simulink model "untitled"  (R2023b)
settings: Solver=ode4  StartTime=0.0  StopTime=100  FixedStep=.02  RelTol=1e-3
values from neighbouring files (symbols this model uses):
  allocation_matrix = [ -0.418379550895652   0.707106781186547   1.000000000000000  -1 ... (first row only)    [Octa_Copter_Parameters.m]
  b_m = 1.645552813e-3    (= 0.001645552813)    [Octa_Copter_Parameters.m]
  d_m = 2.6675567e-3    (= 0.0026675567)    [Octa_Copter_Parameters.m]
  g = 9.81    [Octa_Copter_Parameters.m]
  lx1 = 0.47    [Octa_Copter_Parameters.m]
  lx2 = 0.47    [Octa_Copter_Parameters.m]
  lx3 = 0.47    [Octa_Copter_Parameters.m]
  lx4 = lx1    (= 0.47)    [Octa_Copter_Parameters.m]
  lx5 = 0.47    [Octa_Copter_Parameters.m]
  lx6 = 0.47    [Octa_Copter_Parameters.m]
  lx7 = 0.47    [Octa_Copter_Parameters.m]
  lx8 = lx5    (= 0.47)    [Octa_Copter_Parameters.m]
  ly1 = 0.255    [Octa_Copter_Parameters.m]
  ly2 = 0.255    [Octa_Copter_Parameters.m]
  ly3 = 0.255    [Octa_Copter_Parameters.m]
  ly4 = 0.255    [Octa_Copter_Parameters.m]
  ly5 = 0.548    [Octa_Copter_Parameters.m]
  ly6 = 0.548    [Octa_Copter_Parameters.m]
  ly7 = 0.548    [Octa_Copter_Parameters.m]
  ly8 = 0.548    [Octa_Copter_Parameters.m]
  m = 4.455    [Octa_Copter_Parameters.m]
  omega_nom = sqrt((m*g)/(8*b_m))    [Octa_Copter_Parameters.m]
undefined symbols (not defined in the file or in its folder): L_x_1, L_x_2, sigbuilder_block
libraries: simulink_extras x7, slpidlib x3, shared6dof x1
settings Model: Creator=saifg  LastModifiedBy=saifg
settings SolverCC: ZeroCrossAlgorithm=Adaptive
settings DebuggingCC: IgnoredZcDiagnostic=none

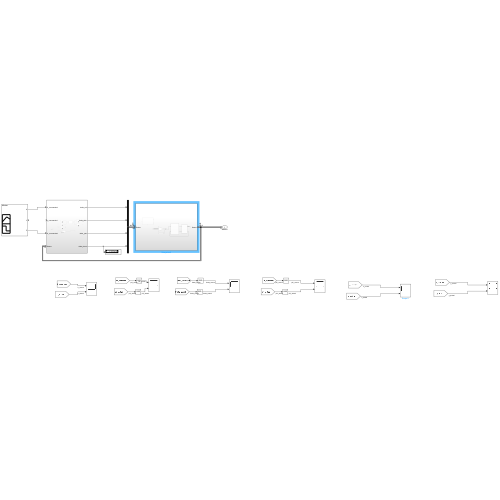
[thumbnail: Simulink's stored preview of the top-level diagram]
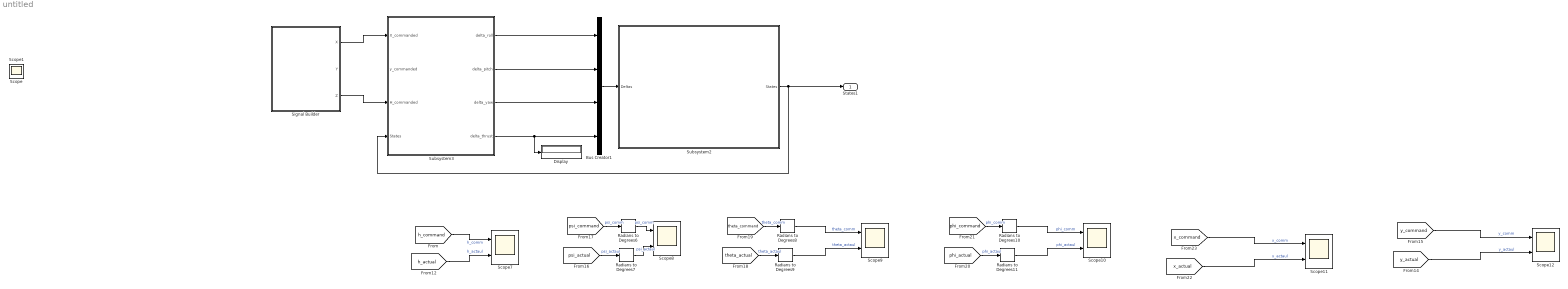
== system untitled ==
  Bus Creator1 : BusCreator  Inputs=4
  Display : Display
  Radians to Degrees{6..11} (6 alike) : simulink_extras/Transformations/Radians to Degrees
  Scope{7..12} (6 alike) : Scope  NumInputPorts=2
  Signal Builder : Subsystem  Tag=STV Subsys  LoadFcn=sigbuilder_block('load');  StartFcn=sigbuilder_block('start');  StopFcn=sigbuilder_block('stop');  ClipboardFcn=sigbuilder_block('clipboard');  mask(Sigbuilder block){tuvar=[0:10]}
      mask help: Simulink:masks:SigbuilderBlock_MD
      mask init:
      | if ~strcmp(get_param(bdroot(gcbh),'SimulationStatus'),'stopped') tuvar = sigbuilder_block('maskInit'); end
      settings: CopyFcn=sigbuilder_block('copy');  DeleteFcn=sigbuilder_block('delete');  ModelCloseFcn=sigbuilder_block('modelClose');  PreSaveFcn=sigbuilder_block('preSave');  PauseFcn=sigbuilder_block('pause');  ContinueFcn=sigbuilder_block('continue');  NameChangeFcn=sigbuilder_block('namechange');  OpenFcn=sigbuilder_block('open',[5.4 36 1141.2 516.6 ]);  CloseFcn=sigbuilder_block('close');
      mask Display: plot(0, 0, 100, 100,[2, 2, 32, 32, 2], [68, 8, 8, 68, 68],[32, 2], [38, 38], [32, 19, 2],[53, 60, 44], [32, 17, 17, 2],[16, 16, 31, 31]);txt = getActiveGroup(gcbh);text(2, 100, txt,'verticalAlignment', 'top');
  Subsystem2 : Subsystem
  Subsystem3 : Subsystem
  States1 : Outport
  Scope : Scope
  Scope1 : Scope
  wires:
  [x_command] -> Scope11/1  "x_comm"
  Bus Creator1/1 -> Subsystem2/1(Deltas)
  [y_command] -> Scope12/1  "y_comm"
  [theta_command] -> Radians to Degrees8/1  "theta_comm"
  [x_actual] -> Scope11/2  "x_actaul"
  [h_actual] -> Scope7/2  "h_actaul"
  Subsystem2/1(States) -> States1/1, Subsystem3/4(States)
  [phi_command] -> Radians to Degrees10/1  "phi_comm"
  Radians to Degrees9/1 -> Scope9/2  "theta_actaul"
  Radians to Degrees10/1 -> Scope10/1  "phi_comm"
  [phi_actual] -> Radians to Degrees11/1  "phi_actaul"
  [theta_actual] -> Radians to Degrees9/1  "theta_actaul"
  [h_command] -> Scope7/1  "h_comm"
  Radians to Degrees11/1 -> Scope10/2  "phi_actaul"
  Radians to Degrees8/1 -> Scope9/1  "theta_comm"
  [psi_actual] -> Radians to Degrees7/1  "psi_actaul"
  Radians to Degrees7/1 -> Scope8/2  "psi_actaul"
  [psi_command] -> Radians to Degrees6/1  "psi_comm"
  Radians to Degrees6/1 -> Scope8/1  "psi_comm"
  [y_actual] -> Scope12/2  "y_actaul"
  Signal Builder/3(Z) -> Subsystem3/3(H_commanded)
  Subsystem3/4(delta_thrust) -> Bus Creator1/4, Display/1
  Subsystem3/1(delta_roll) -> Bus Creator1/1
  Subsystem3/2(delta_pitch) -> Bus Creator1/2
  Subsystem3/3(delta_yaw) -> Bus Creator1/3
  Signal Builder/1(X) -> Subsystem3/1(X_commanded)

== system untitled/Signal Builder ==
  Demux : Demux  Tag=STV Demux  Outputs=3
      settings: DisplayOption=none
  FromWs : FromWorkspace  Tag=STV FromWs  VariableName=tuvar
      SigBuilderData=|
      | common.afterFinalStr = 'Extrapolate'
      | common.sampleTime = 0
      | dataSet.timeRange = [0 2000]
      | dataSet.name = 'Mission'
      | sbobj.Name = 'Signal Builder'
      | sbobj.Groups.Name = 'Mission'
      | sbobj.Groups.Signals(1).Name = 'X'
      | sbobj.Groups.Signals(1).XData = [0 20.1 20.1 66.55 66.55 2000]
      | sbobj.Groups.Signals(1).YData = [0 0 1 1 0 0]
      | sbobj.Groups.Signals(2).Name = 'Y'
      | sbobj.Groups.Signals(2).XData = [0 24 24 64.3 64.3 2000]
      | sbobj.Groups.Signals(2).YData = [0 0 1 1 0 0]
      | sbobj.Groups.Signals(3).Name = 'Z'
      | sbobj.Groups.Signals(3).XData = [0 2000]
      | sbobj.Groups.Signals(3).YData = [10 10]
      | sbobj.Groups.TimeRange = [0 2000]
  X : Outport  Tag=STV Outport
  Y : Outport  Tag=STV Outport  Port=2
  Z : Outport  Tag=STV Outport  Port=3
  wires:
  FromWs/1 -> Demux/1
  Demux/1 -> X/1
  Demux/2 -> Y/1
  Demux/3 -> Z/1

== system untitled/Subsystem2 ==
  Deltas : Inport
  Add : Sum
  Allocation Matrix : Gain  Gain=allocation_matrix  Multiplication=Matrix(K*u)
  Constant4 : Constant  Value=omega_nom*ones(8,1)
  Forces & Moment : Subsystem
  Subsystem : Subsystem
  Subsystem2 : Subsystem  Commented=on
      settings: PortSchema="{\"entries\":[{\"content\":{\"sides\":[{\"content\":{\"connectorIds\":[\"In1\"]},\"type\":\"ConnectorPlacement.EquallySpacedRectSide\",\"uuid\":\"5560b1ac-f730-4650-bcff-b5f0178619bd\"},{\"content\":{\"connectorIds\":[\"Out1\",\"Out2\"],\"side\":\"RIGHT\"},\"type\":\"ConnectorPlacement.EquallySpacedRectSide\",\"uuid\":\"fca2ce35-7b68-4ca4-aed6-61d3950c0b58\"},{\"content\":{\"side\":\"TOP\"},\"type\":\"ConnectorPlacement.EquallySpacedRectSide\",\"uuid\":\"dce7e5b3-bb13-4631-9d75-8f7199e09c42\"},{\"content\":{\"connectorIds\":[\"In2\"],\"side\":\"BOTTOM\"},\"type\":\"ConnectorPlacement.EquallySpacedRectSide\",\"uuid\":\"cf384071-4b3c-41fd-9fcc-1c3085bccb35\"}]},\"type\":\"ConnectorPlacement.EquallySpacedConnector\",\"uuid\":\"aa4e0d9e-47a4-41f4-8eed-feabe2aa2793\"}],\"packageUris\":[\"http://schema.mathworks.com/mf0/Connector/R2020b\"],\"version\":\"1.0\"}"
  States : Outport
  wires:
  Subsystem/1(States) -> States/1
  Add/1 -> Forces & Moment/1(omegas)
  Constant4/1 -> Add/2
  Subsystem/2(DCM) -> Forces & Moment/2(DCM)
  Allocation Matrix/1 -> Add/1
  Forces & Moment/2(Moment) -> Subsystem/2(Moments)
  Deltas/1 -> Allocation Matrix/1
  Forces & Moment/1(Force) -> Subsystem/1(Forces)

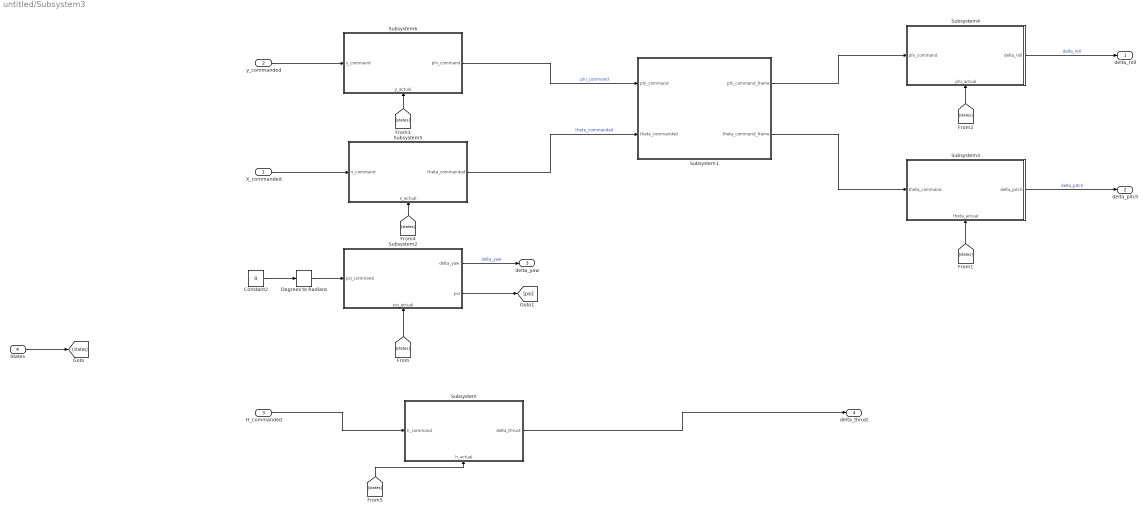
== system untitled/Subsystem3 ==
  X_commanded : Inport
  y_commanded : Inport  Port=2
  H_commanded : Inport  Port=3
  States : Inport  Port=4
  Constant2 : Constant  Value=0
  Degrees to Radians : simulink_extras/Transformations/Degrees to Radians
  Subsystem : Subsystem
      settings: PortSchema="{\"entries\":[{\"content\":{\"sides\":[{\"content\":{\"connectorIds\":[\"In1\"]},\"type\":\"ConnectorPlacement.EquallySpacedRectSide\",\"uuid\":\"f70ca49b-3fc5-44f8-8cd5-c7690505358d\"},{\"content\":{\"connectorIds\":[\"Out1\"],\"side\":\"RIGHT\"},\"type\":\"ConnectorPlacement.EquallySpacedRectSide\",\"uuid\":\"144fa0cf-5b2f-4865-9591-bfb41d20b3c6\"},{\"content\":{\"side\":\"TOP\"},\"type\":\"ConnectorPlacement.EquallySpacedRectSide\",\"uuid\":\"1b5c934e-468c-402b-9c74-0dd4bd7d6b0a\"},{\"content\":{\"connectorIds\":[\"In2\"],\"side\":\"BOTTOM\"},\"type\":\"ConnectorPlacement.EquallySpacedRectSide\",\"uuid\":\"b6ed394a-e2c0-4d90-8876-cfec3c3b0be2\"}]},\"type\":\"ConnectorPlacement.EquallySpacedConnector\",\"uuid\":\"8d96b359-1377-43c1-9baa-eb90b377e467\"}],\"packageUris\":[\"http://schema.mathworks.com/mf0/Connector/R2020b\"],\"version\":\"1.0\"}"
  Subsystem1 : Subsystem
  Subsystem2 : Subsystem
      settings: PortSchema="{\"entries\":[{\"content\":{\"sides\":[{\"content\":{\"connectorIds\":[\"In1\"]},\"type\":\"ConnectorPlacement.EquallySpacedRectSide\",\"uuid\":\"f70ca49b-3fc5-44f8-8cd5-c7690505358d\"},{\"content\":{\"connectorIds\":[\"Out1\",\"Out2\"],\"side\":\"RIGHT\"},\"type\":\"ConnectorPlacement.EquallySpacedRectSide\",\"uuid\":\"144fa0cf-5b2f-4865-9591-bfb41d20b3c6\"},{\"content\":{\"side\":\"TOP\"},\"type\":\"ConnectorPlacement.EquallySpacedRectSide\",\"uuid\":\"1b5c934e-468c-402b-9c74-0dd4bd7d6b0a\"},{\"content\":{\"connectorIds\":[\"In2\"],\"side\":\"BOTTOM\"},\"type\":\"ConnectorPlacement.EquallySpacedRectSide\",\"uuid\":\"b6ed394a-e2c0-4d90-8876-cfec3c3b0be2\"}]},\"type\":\"ConnectorPlacement.EquallySpacedConnector\",\"uuid\":\"8d96b359-1377-43c1-9baa-eb90b377e467\"}],\"packageUris\":[\"http://schema.mathworks.com/mf0/Connector/R2020b\"],\"version\":\"1.0\"}"
  Subsystem3 : Subsystem
      settings: PortSchema="{\"entries\":[{\"content\":{\"sides\":[{\"content\":{\"connectorIds\":[\"In1\"]},\"type\":\"ConnectorPlacement.EquallySpacedRectSide\",\"uuid\":\"f70ca49b-3fc5-44f8-8cd5-c7690505358d\"},{\"content\":{\"connectorIds\":[\"Out1\"],\"side\":\"RIGHT\"},\"type\":\"ConnectorPlacement.EquallySpacedRectSide\",\"uuid\":\"144fa0cf-5b2f-4865-9591-bfb41d20b3c6\"},{\"content\":{\"side\":\"TOP\"},\"type\":\"ConnectorPlacement.EquallySpacedRectSide\",\"uuid\":\"1b5c934e-468c-402b-9c74-0dd4bd7d6b0a\"},{\"content\":{\"connectorIds\":[\"In2\"],\"side\":\"BOTTOM\"},\"type\":\"ConnectorPlacement.EquallySpacedRectSide\",\"uuid\":\"b6ed394a-e2c0-4d90-8876-cfec3c3b0be2\"}]},\"type\":\"ConnectorPlacement.EquallySpacedConnector\",\"uuid\":\"8d96b359-1377-43c1-9baa-eb90b377e467\"}],\"packageUris\":[\"http://schema.mathworks.com/mf0/Connector/R2020b\"],\"version\":\"1.0\"}"
  Subsystem4 : Subsystem
      settings: PortSchema="{\"entries\":[{\"content\":{\"sides\":[{\"content\":{\"connectorIds\":[\"In1\"]},\"type\":\"ConnectorPlacement.EquallySpacedRectSide\",\"uuid\":\"f70ca49b-3fc5-44f8-8cd5-c7690505358d\"},{\"content\":{\"connectorIds\":[\"Out1\"],\"side\":\"RIGHT\"},\"type\":\"ConnectorPlacement.EquallySpacedRectSide\",\"uuid\":\"144fa0cf-5b2f-4865-9591-bfb41d20b3c6\"},{\"content\":{\"side\":\"TOP\"},\"type\":\"ConnectorPlacement.EquallySpacedRectSide\",\"uuid\":\"1b5c934e-468c-402b-9c74-0dd4bd7d6b0a\"},{\"content\":{\"connectorIds\":[\"In2\"],\"side\":\"BOTTOM\"},\"type\":\"ConnectorPlacement.EquallySpacedRectSide\",\"uuid\":\"b6ed394a-e2c0-4d90-8876-cfec3c3b0be2\"}]},\"type\":\"ConnectorPlacement.EquallySpacedConnector\",\"uuid\":\"8d96b359-1377-43c1-9baa-eb90b377e467\"}],\"packageUris\":[\"http://schema.mathworks.com/mf0/Connector/R2020b\"],\"version\":\"1.0\"}"
  Subsystem5 : Subsystem
      settings: PortSchema="{\"entries\":[{\"content\":{\"sides\":[{\"content\":{\"connectorIds\":[\"In1\"]},\"type\":\"ConnectorPlacement.EquallySpacedRectSide\",\"uuid\":\"f70ca49b-3fc5-44f8-8cd5-c7690505358d\"},{\"content\":{\"connectorIds\":[\"Out1\"],\"side\":\"RIGHT\"},\"type\":\"ConnectorPlacement.EquallySpacedRectSide\",\"uuid\":\"144fa0cf-5b2f-4865-9591-bfb41d20b3c6\"},{\"content\":{\"side\":\"TOP\"},\"type\":\"ConnectorPlacement.EquallySpacedRectSide\",\"uuid\":\"1b5c934e-468c-402b-9c74-0dd4bd7d6b0a\"},{\"content\":{\"connectorIds\":[\"In2\"],\"side\":\"BOTTOM\"},\"type\":\"ConnectorPlacement.EquallySpacedRectSide\",\"uuid\":\"b6ed394a-e2c0-4d90-8876-cfec3c3b0be2\"}]},\"type\":\"ConnectorPlacement.EquallySpacedConnector\",\"uuid\":\"8d96b359-1377-43c1-9baa-eb90b377e467\"}],\"packageUris\":[\"http://schema.mathworks.com/mf0/Connector/R2020b\"],\"version\":\"1.0\"}"
  Subsystem6 : Subsystem
      settings: PortSchema="{\"entries\":[{\"content\":{\"sides\":[{\"content\":{\"connectorIds\":[\"In1\"]},\"type\":\"ConnectorPlacement.EquallySpacedRectSide\",\"uuid\":\"f70ca49b-3fc5-44f8-8cd5-c7690505358d\"},{\"content\":{\"connectorIds\":[\"Out1\"],\"side\":\"RIGHT\"},\"type\":\"ConnectorPlacement.EquallySpacedRectSide\",\"uuid\":\"144fa0cf-5b2f-4865-9591-bfb41d20b3c6\"},{\"content\":{\"side\":\"TOP\"},\"type\":\"ConnectorPlacement.EquallySpacedRectSide\",\"uuid\":\"1b5c934e-468c-402b-9c74-0dd4bd7d6b0a\"},{\"content\":{\"connectorIds\":[\"In2\"],\"side\":\"BOTTOM\"},\"type\":\"ConnectorPlacement.EquallySpacedRectSide\",\"uuid\":\"b6ed394a-e2c0-4d90-8876-cfec3c3b0be2\"}]},\"type\":\"ConnectorPlacement.EquallySpacedConnector\",\"uuid\":\"8d96b359-1377-43c1-9baa-eb90b377e467\"}],\"packageUris\":[\"http://schema.mathworks.com/mf0/Connector/R2020b\"],\"version\":\"1.0\"}"
  delta_roll : Outport
  delta_pitch : Outport  Port=2
  delta_yaw : Outport  Port=3
  delta_thrust : Outport  Port=4
  wires:
  Constant2/1 -> Degrees to Radians/1
  Degrees to Radians/1 -> Subsystem2/1(psi_command)
  X_commanded/1 -> Subsystem5/1(x_command)
  Subsystem3/1(delta_pitch) -> delta_pitch/1  "delta_pitch"
  Subsystem2/1(delta_yaw) -> delta_yaw/1  "delta_yaw"
  Subsystem/1(delta_thrust) -> delta_thrust/1
  Subsystem4/1(delta_roll) -> delta_roll/1  "delta_roll"
  y_commanded/1 -> Subsystem6/1(y_command)
  States/1 -> [states]
  [states] -> Subsystem2/2(psi_actual)
  Subsystem2/2(psi) -> [psi]
  [states] -> Subsystem3/2(theta_actual)
  [states] -> Subsystem4/2(phi_actual)
  [states] -> Subsystem6/2(y_actual)
  [states] -> Subsystem5/2(x_actual)
  H_commanded/1 -> Subsystem/1(h_command)
  [states] -> Subsystem/2(h_actual)
  Subsystem1/1(phi_command_frame) -> Subsystem4/1(phi_command)
  Subsystem1/2(theta_command_frame) -> Subsystem3/1(theta_command)
  Subsystem6/1(phi_command) -> Subsystem1/1(phi_command)  "phi_command"
  Subsystem5/1(theta_commanded) -> Subsystem1/2(theta_commanded)  "theta_commanded"

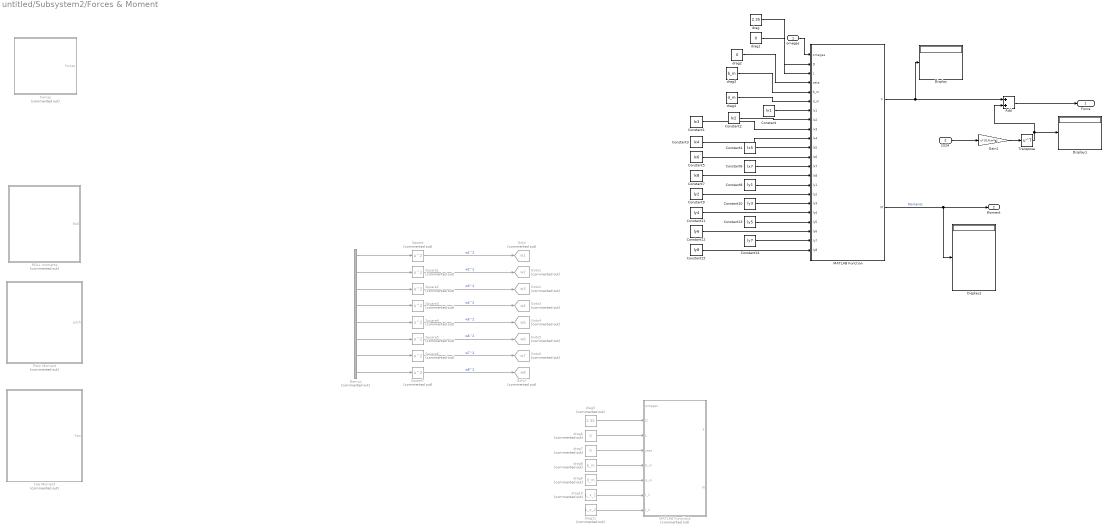
== system untitled/Subsystem2/Forces & Moment ==
  omegas : Inport
  DCM : Inport  Port=2
  Add : Sum
  Constant : Constant  Value=lx1
  Constant1 : Constant  Value=lx3
  Constant10 : Constant  Value=ly3
  Constant11 : Constant  Value=ly4
  Constant12 : Constant  Value=ly6
  Constant13 : Constant  Value=ly5
  Constant14 : Constant  Value=ly7
  Constant15 : Constant  Value=ly8
  Constant2 : Constant  Value=lx2
  Constant3 : Constant  Value=lx4
  Constant4 : Constant  Value=lx5
  Constant5 : Constant  Value=lx6
  Constant6 : Constant  Value=lx7
  Constant7 : Constant  Value=lx8
  Constant8 : Constant  Value=ly1
  Constant9 : Constant  Value=ly2
  Demux : Demux  Commented=on  Outputs=8
  Display : Display
  Display1 : Display
  Display2 : Display
  Forces : Subsystem  Commented=on
  Gain1 : Gain  Gain=[0;0;m*g]  Multiplication=Matrix(u*K)
  Goto : Goto  Commented=on  GotoTag=w1  TagVisibility=global
  Goto1 : Goto  Commented=on  GotoTag=w2  TagVisibility=global
  Goto2 : Goto  Commented=on  GotoTag=w3  TagVisibility=global
  Goto3 : Goto  Commented=on  GotoTag=w4  TagVisibility=global
  Goto4 : Goto  Commented=on  GotoTag=w5  TagVisibility=global
  Goto5 : Goto  Commented=on  GotoTag=w6  TagVisibility=global
  Goto6 : Goto  Commented=on  GotoTag=w7  TagVisibility=global
  Goto7 : Goto  Commented=on  GotoTag=w8  TagVisibility=global
  MATLAB Function : MATLAB Function  TreatAsAtomicUnit=on
  MATLAB Function1 : MATLAB Function  Commented=on  TreatAsAtomicUnit=on
  Pitch Moment : Subsystem  Commented=on
  ROLL moments : Subsystem  Commented=on
  Square{,1..7} (8 alike) : Math  Commented=on  Operator=square
  Transpose : Math  Operator=transpose
  Yaw Moment : Subsystem  Commented=on
  drag : Constant  Value=2.35
  drag1 : Constant  Value=0
  drag10 : Constant  Commented=on  Value=L_x_1
  drag11 : Constant  Commented=on  Value=L_x_2
  drag2 : Constant  Value=0
  drag3 : Constant  Value=b_m
  drag4 : Constant  Value=d_m
  drag5 : Constant  Commented=on  Value=2.35
  drag6 : Constant  Commented=on  Value=0
  drag7 : Constant  Commented=on  Value=0
  drag8 : Constant  Commented=on  Value=b_m
  drag9 : Constant  Commented=on  Value=d_m
  Force : Outport
  Moment : Outport  Port=2
  wires:
  Square/1 -> Goto/1  "w1^2"
  Square1/1 -> Goto1/1  "w2^2"
  Square2/1 -> Goto2/1  "w3^2"
  Square3/1 -> Goto3/1  "w4^2"
  Square4/1 -> Goto4/1  "w5^2"
  Square5/1 -> Goto5/1  "w6^2"
  Square6/1 -> Goto6/1  "w7^2"
  Square7/1 -> Goto7/1  "w8^2"
  Demux/1 -> Square/1
  Demux/2 -> Square1/1
  Demux/3 -> Square2/1
  Demux/4 -> Square3/1
  Demux/5 -> Square4/1
  Demux/6 -> Square5/1
  Demux/7 -> Square6/1
  Demux/8 -> Square7/1
  Constant15/1 -> MATLAB Function/22(ly8)
  Constant2/1 -> MATLAB Function/8(lx2)
  Constant11/1 -> MATLAB Function/18(ly4)
  drag4/1 -> MATLAB Function/6(d_m)
  Gain1/1 -> Transpose/1
  Constant12/1 -> MATLAB Function/20(ly6)
  Constant9/1 -> MATLAB Function/16(ly2)
  Constant13/1 -> MATLAB Function/19(ly5)
  Constant10/1 -> MATLAB Function/17(ly3)
  Constant/1 -> MATLAB Function/7(lx1)
  Constant3/1 -> MATLAB Function/10(lx4)
  drag3/1 -> MATLAB Function/5(b_m)
  Constant1/1 -> MATLAB Function/9(lx3)
  Constant5/1 -> MATLAB Function/12(lx6)
  Constant8/1 -> MATLAB Function/15(ly1)
  DCM/1 -> Gain1/1
  drag1/1 -> MATLAB Function/3(L)
  Constant14/1 -> MATLAB Function/21(ly7)
  drag2/1 -> MATLAB Function/4(ceta)
  Transpose/1 -> Add/2, Display1/1
  Add/1 -> Force/1
  Constant4/1 -> MATLAB Function/11(lx5)
  Constant6/1 -> MATLAB Function/13(lx7)
  Constant7/1 -> MATLAB Function/14(lx8)
  drag/1 -> MATLAB Function/2(D)
  drag11/1 -> MATLAB Function1/8(l_2)
  drag8/1 -> MATLAB Function1/5(b_m)
  drag6/1 -> MATLAB Function1/3(L)
  drag5/1 -> MATLAB Function1/2(D)
  drag9/1 -> MATLAB Function1/6(d_m)
  drag10/1 -> MATLAB Function1/7(l_1)
  drag7/1 -> MATLAB Function1/4(ceta)
  omegas/1 -> MATLAB Function/1(omegas)
  MATLAB Function/1(F) -> Display/1, Add/1
  MATLAB Function/2(M) -> Moment/1, Display2/1  "Moments"

== system untitled/Subsystem2/Subsystem ==
  Forces : Inport
  Moments : Inport  Port=2
  6DOF (Euler Angles) : shared6dof/6DOF (Euler Angles)  units=Metric (MKS)  mtype=Fixed  rep=Euler Angles  xme_0=[0 0 -1]  Vm_0=[0 0 0]  eul_0=[0 0 0]  pm_0=[0 0 0]  mass_0=m  mass_e=0.5  mass_f=2.0  inertia=I  inertia_e=eye(3)  inertia_f=2*eye(3)  k_quat=1.0  vre_flag=on  abi_flag=off  aMode=0  xme_statename=''  Vm_statename=''  eul_statename=''  quat_statename=''  pm_statename=''  mass_statename=''
  Bus Creator : BusCreator  Inputs=12
  Demux{,1..2,4} (4 alike) : Demux  Outputs=3
  States : Outport
  DCM : Outport  Port=2
  tag scope: z=global
  wires:
  6DOF (Euler Angles)/4 -> DCM/1  "DCM"
  Forces/1 -> 6DOF (Euler Angles)/1
  Demux1/3 -> Bus Creator/6  "epsi"
  6DOF (Euler Angles)/5 -> Demux4/1
  Moments/1 -> 6DOF (Euler Angles)/2
  6DOF (Euler Angles)/2 -> Demux/1
  Demux/1 -> Bus Creator/1  "X"
  6DOF (Euler Angles)/3 -> Demux1/1
  6DOF (Euler Angles)/6 -> Demux2/1
  Demux/2 -> Bus Creator/2  "Y"
  Demux/3 -> [z], Bus Creator/3  "Z"
  Demux1/1 -> Bus Creator/4  "phi"
  Demux1/2 -> Bus Creator/5  "theta"
  Demux4/1 -> Bus Creator/7  "Vx_b"
  Demux4/2 -> Bus Creator/8  "Vy_b"
  Demux4/3 -> Bus Creator/9  "vz_b"
  Demux2/1 -> Bus Creator/10  "p"
  Demux2/2 -> Bus Creator/11  "q"
  Demux2/3 -> Bus Creator/12  "r"
  Bus Creator/1 -> States/1

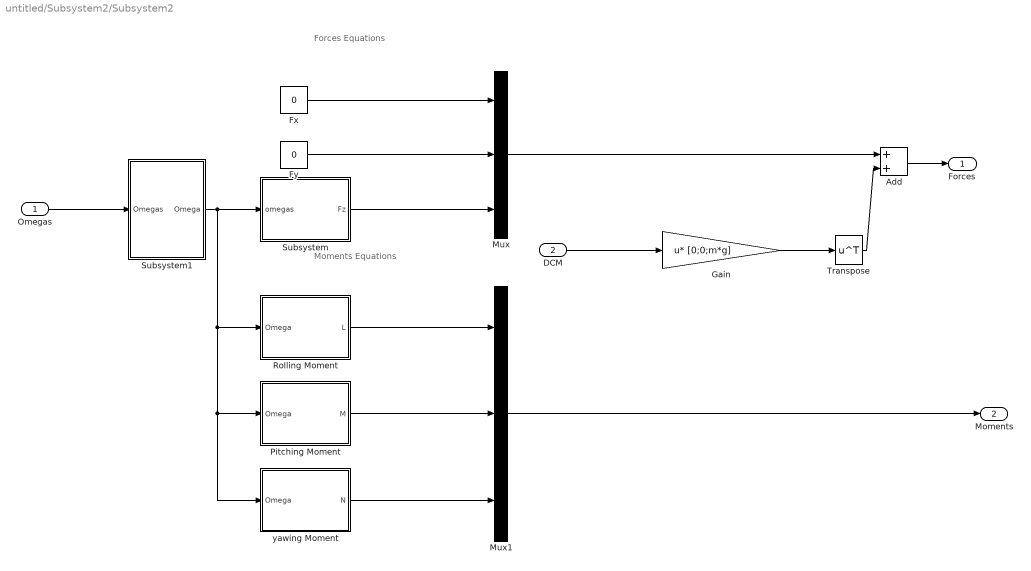
== system untitled/Subsystem2/Subsystem2 ==
  note: Forces Equations
  note: Moments Equations
  Omegas : Inport
  DCM : Inport  Port=2
  Add : Sum
  Fx : Constant  Value=0
  Fy : Constant  Value=0
  Gain : Gain  Gain=[0;0;m*g]  Multiplication=Matrix(u*K)
  Mux : Mux  Inputs=3
  Mux1 : Mux  Inputs=3
  Pitching Moment : Subsystem
  Rolling Moment : Subsystem
  Subsystem : Subsystem
  Subsystem1 : Subsystem
  Transpose : Math  Operator=transpose
  yawing Moment : Subsystem
  Forces : Outport
  Moments : Outport  Port=2
  wires:
  Fy/1 -> Mux/2
  Pitching Moment/1(M) -> Mux1/2
  Omegas/1 -> Subsystem1/1(Omegas)
  Fx/1 -> Mux/1
  Subsystem1/1(Omega) -> yawing Moment/1(Omega), Pitching Moment/1(Omega), Rolling Moment/1(Omega), Subsystem/1(omegas)
  Subsystem/1(Fz) -> Mux/3
  Rolling Moment/1(L) -> Mux1/1
  yawing Moment/1(N) -> Mux1/3
  Mux1/1 -> Moments/1
  Gain/1 -> Transpose/1
  Mux/1 -> Add/1
  Transpose/1 -> Add/2
  Add/1 -> Forces/1
  DCM/1 -> Gain/1

== system untitled/Subsystem3/Subsystem ==
  h_command : Inport
  h_actual : Inport  Port=2
  Bus Selector : BusSelector  OutputSignals=Z
  Derivative : Derivative
  Gain1 : Gain  Gain=-1
  Kd : Gain  Gain=89
  PID Controller : slpidlib/PID Controller  Controller=PI  Form=Parallel  TimeDomain=Continuous-time  UseExternalTs=off  SampleTime=-1  IntegratorMethod=Forward Euler  FilterMethod=Forward Euler  ControllerParametersSource=internal  P=50  I=12  UseKiTs=off  D=0  N=100  UseFilter=on  TunerSelectOption=Transfer Function Based (PID Tuner App)  InitialConditionSource=internal  InitialConditionForIntegrator=0  InitialConditionForFilter=0  DifferentiatorICPrevScaledInput=0  ExternalReset=none  TrackingMode=off  Kt=1  LimitOutput=off  SatLimitsSource=internal  UpperSaturationLimit=inf  LowerSaturationLimit=-inf  LinearizeAsGain=on  AntiWindupMode=none  Kb=1  LimitIntegrator=off  UpperIntegratorSaturationLimit=inf  LowerIntegratorSaturationLimit=-inf  POutMin=[]  POutMax=[]  IOutMin=[]  IOutMax=[]  DOutMin=[]  DOutMax=[]  NOutMin=[]  NOutMax=[]  SumOutMin=[]  SumOutMax=[]  SaturationOutMin=[]  SaturationOutMax=[]  PParamMin=[]  PParamMax=[]  IParamMin=[]  IParamMax=[]  DParamMin=[]  DParamMax=[]  NParamMin=[]  NParamMax=[]  KbParamMin=[]  KbParamMax=[]  KtParamMin=[]  KtParamMax=[]  KbOutMin=[]  KbOutMax=[]  KtOutMin=[]  KtOutMax=[]  IntegratorOutMin=[]  IntegratorOutMax=[]  FilterOutMin=[]  FilterOutMax=[]  SumI1OutMin=[]  SumI1OutMax=[]  SumI2OutMin=[]  SumI2OutMax=[]  SumI3OutMin=[]  SumI3OutMax=[]  SumI4OutMin=[]  SumI4OutMax=[]  SumDOutMin=[]  SumDOutMax=[]  DifferentiatorOutMin=[]  DifferentiatorOutMax=[]  FilterDiffOutCoefMin=[]  FilterDiffOutCoefMax=[]  ReciprocalOutMin=[]  ReciprocalOutMax=[]  SumDenOutMin=[]  SumDenOutMax=[]  SumNumOutMin=[]  SumNumOutMax=[]  DivideOutMin=[]  DivideOutMax=[]  UdiffTsProdOutMin=[]  UdiffTsProdOutMax=[]  NTsProdOutMin=[]  NTsProdOutMax=[]  UintegralTsProdOutMin=[]  UintegralTsProdOutMax=[]  UngainTsProdOutMin=[]  UngainTsProdOutMax=[]  ClampingZeroOutDataTypeStr=Inherit: Inherit via back propagation  ClampingZeroOutMin=[]  ClampingZeroOutMax=[]  FilterDenConstantOutDataTypeStr=Inherit: Inherit via back propagation  FilterDenConstantOutMin=[]  FilterDenConstantOutMax=[]  PCopyOutDataTypeStr=Inherit: Inherit via back propagation  PCopyOutMin=[]  PCopyOutMax=[]  NCopyOutDataTypeStr=Inherit: Inherit via back propagation  NCopyOutMin=[]  NCopyOutMax=[]  IntegratorContinuousStateAttributes=''  IntegratorStateMustResolveToSignalObject=off  IntegratorRTWStateStorageClass=Auto  FilterContinuousStateAttributes=''  FilterStateMustResolveToSignalObject=off  FilterRTWStateStorageClass=Auto  ParallelPVariant=InternalParameters  IdealPVariant=Disabled  IVariant=InternalParameters  DVariant=Disabled  IntegratorVariant=Continuous  SatVariant=Disabled  AWVariant=Passthrough  PCopyVariant=Disabled  TRVariant=Disabled  FdbkBlocksVariant=Forward  IdealPFdbkVariant=Disabled  SatFdbkVariant=Disabled  DerivativeFilterVariant=Disabled  NVariant=Disabled  NCopyVariant=Disabled_SignalSpec  FilterICVariant=Disabled  IntegratorICVariant=InternalICs  ExternalResetVariant=Disabled  TRSumVariant=Passthrough  SumFdbkVariant=Disabled  SumVariant=Sum_PI  TsampFilterVariant=InternalTs  TsampNgainVariant=Passthrough  TsampIntegralVariant=Disabled_SignalSpec  ExternalSaturationOutDataTypeStr=Inherit: Same as second input
  Sum : Sum  Inputs=|++
  Sum1 : Sum  Inputs=|++
  delta_thrust : Outport
  tag scope: h_actual=global, h_command=global
  wires:
  h_actual/1 -> Bus Selector/1
  Bus Selector/1 -> Kd/1, Sum/2, Gain1/1  "<Z>"
  h_command/1 -> [h_command], Sum/1
  Gain1/1 -> [h_actual]
  Kd/1 -> Derivative/1
  PID Controller/1 -> Sum1/1
  Sum/1 -> PID Controller/1
  Derivative/1 -> Sum1/2
  Sum1/1 -> delta_thrust/1

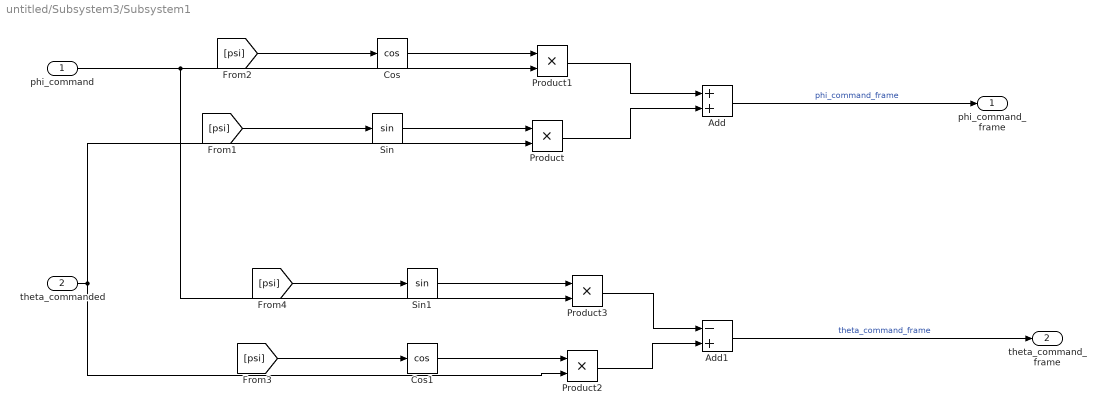
== system untitled/Subsystem3/Subsystem1 ==
  phi_command : Inport
  theta_commanded : Inport  Port=2
  Add : Sum
  Add1 : Sum  Inputs=-+
  Cos : Trigonometry  Operator=cos
  Cos1 : Trigonometry  Operator=cos
  Product{,1..3} (4 alike) : Product
  Sin : Trigonometry
  Sin1 : Trigonometry
  phi_command_frame : Outport
  theta_command_frame : Outport  Port=2
  wires:
  [psi] -> Cos/1
  theta_commanded/1 -> Product/2, Product2/2
  Sin1/1 -> Product3/1
  Sin/1 -> Product/1
  Product1/1 -> Add/1
  [psi] -> Cos1/1
  phi_command/1 -> Product3/2, Product1/2
  [psi] -> Sin/1
  Cos1/1 -> Product2/1
  Product/1 -> Add/2
  Product3/1 -> Add1/1
  Product2/1 -> Add1/2
  Cos/1 -> Product1/1
  Add1/1 -> theta_command_frame/1  "theta_command_frame"
  Add/1 -> phi_command_frame/1  "phi_command_frame"
  [psi] -> Sin1/1

== system untitled/Subsystem3/Subsystem2 ==
  psi_command : Inport
  psi_actual : Inport  Port=2
  Bus Selector : BusSelector  OutputSignals=epsi
  Derivative : Derivative
  Gain : Gain  Gain=60
  Gain1 : Gain  Gain=36
  Sum : Sum  Inputs=|+-
  Sum1 : Sum  Inputs=|+-
  delta_yaw : Outport
  psi : Outport  Port=2
  tag scope: psi_actual=global, psi_command=global
  wires:
  psi_command/1 -> Sum/1, [psi_command]
  Bus Selector/1 -> Derivative/1, Sum/2, psi/1, [psi_actual]  "<epsi>"
  psi_actual/1 -> Bus Selector/1
  Sum/1 -> Gain/1  "error"
  Sum1/1 -> delta_yaw/1
  Gain/1 -> Sum1/1
  Derivative/1 -> Gain1/1
  Gain1/1 -> Sum1/2

== system untitled/Subsystem3/Subsystem3 ==
  theta_command : Inport
  theta_actual : Inport  Port=2
  Bus Selector : BusSelector  OutputSignals=theta
  PID Controller : slpidlib/PID Controller  Controller=PD  Form=Parallel  TimeDomain=Continuous-time  UseExternalTs=off  SampleTime=-1  IntegratorMethod=Forward Euler  FilterMethod=Forward Euler  ControllerParametersSource=internal  P=7  I=57.479  UseKiTs=off  D=10  N=100  UseFilter=on  TunerSelectOption=Transfer Function Based (PID Tuner App)  InitialConditionSource=internal  InitialConditionForIntegrator=0  InitialConditionForFilter=0  DifferentiatorICPrevScaledInput=0  ExternalReset=none  TrackingMode=off  Kt=1  LimitOutput=off  SatLimitsSource=internal  UpperSaturationLimit=inf  LowerSaturationLimit=-inf  LinearizeAsGain=on  AntiWindupMode=none  Kb=1  LimitIntegrator=off  UpperIntegratorSaturationLimit=inf  LowerIntegratorSaturationLimit=-inf  POutMin=[]  POutMax=[]  IOutMin=[]  IOutMax=[]  DOutMin=[]  DOutMax=[]  NOutMin=[]  NOutMax=[]  SumOutMin=[]  SumOutMax=[]  SaturationOutMin=[]  SaturationOutMax=[]  PParamMin=[]  PParamMax=[]  IParamMin=[]  IParamMax=[]  DParamMin=[]  DParamMax=[]  NParamMin=[]  NParamMax=[]  KbParamMin=[]  KbParamMax=[]  KtParamMin=[]  KtParamMax=[]  KbOutMin=[]  KbOutMax=[]  KtOutMin=[]  KtOutMax=[]  IntegratorOutMin=[]  IntegratorOutMax=[]  FilterOutMin=[]  FilterOutMax=[]  SumI1OutMin=[]  SumI1OutMax=[]  SumI2OutMin=[]  SumI2OutMax=[]  SumI3OutMin=[]  SumI3OutMax=[]  SumI4OutMin=[]  SumI4OutMax=[]  SumDOutMin=[]  SumDOutMax=[]  DifferentiatorOutMin=[]  DifferentiatorOutMax=[]  FilterDiffOutCoefMin=[]  FilterDiffOutCoefMax=[]  ReciprocalOutMin=[]  ReciprocalOutMax=[]  SumDenOutMin=[]  SumDenOutMax=[]  SumNumOutMin=[]  SumNumOutMax=[]  DivideOutMin=[]  DivideOutMax=[]  UdiffTsProdOutMin=[]  UdiffTsProdOutMax=[]  NTsProdOutMin=[]  NTsProdOutMax=[]  UintegralTsProdOutMin=[]  UintegralTsProdOutMax=[]  UngainTsProdOutMin=[]  UngainTsProdOutMax=[]  ClampingZeroOutDataTypeStr=Inherit: Inherit via back propagation  ClampingZeroOutMin=[]  ClampingZeroOutMax=[]  FilterDenConstantOutDataTypeStr=Inherit: Inherit via back propagation  FilterDenConstantOutMin=[]  FilterDenConstantOutMax=[]  PCopyOutDataTypeStr=Inherit: Inherit via back propagation  PCopyOutMin=[]  PCopyOutMax=[]  NCopyOutDataTypeStr=Inherit: Inherit via back propagation  NCopyOutMin=[]  NCopyOutMax=[]  IntegratorContinuousStateAttributes=''  IntegratorStateMustResolveToSignalObject=off  IntegratorRTWStateStorageClass=Auto  FilterContinuousStateAttributes=''  FilterStateMustResolveToSignalObject=off  FilterRTWStateStorageClass=Auto  ParallelPVariant=InternalParameters  IdealPVariant=Disabled  IVariant=Disabled  DVariant=InternalParameters  IntegratorVariant=Disabled  SatVariant=Disabled  AWVariant=Disabled  PCopyVariant=Disabled  TRVariant=Disabled  FdbkBlocksVariant=Forward  IdealPFdbkVariant=Disabled  SatFdbkVariant=Disabled  DerivativeFilterVariant=ContFilter  NVariant=InternalParameters  NCopyVariant=Disabled  FilterICVariant=InternalICsFilter  IntegratorICVariant=Disabled  ExternalResetVariant=Disabled  TRSumVariant=Passthrough  SumFdbkVariant=Disabled  SumVariant=Sum_PD  TsampFilterVariant=InternalTs  TsampNgainVariant=Passthrough  TsampIntegralVariant=Disabled_SignalSpec  ExternalSaturationOutDataTypeStr=Inherit: Same as second input
  Sum : Sum  Inputs=|+-
  delta_pitch : Outport
  tag scope: theta_actual=global, theta_command=global
  wires:
  theta_actual/1 -> Bus Selector/1
  Bus Selector/1 -> [theta_actual], Sum/2  "<theta>"
  theta_command/1 -> [theta_command], Sum/1
  Sum/1 -> PID Controller/1  "error"
  PID Controller/1 -> delta_pitch/1

== system untitled/Subsystem3/Subsystem4 ==
  phi_command : Inport
  phi_actual : Inport  Port=2
  Bus Selector : BusSelector  OutputSignals=phi
  PID Controller1 : slpidlib/PID Controller  Controller=PD  Form=Parallel  TimeDomain=Continuous-time  UseExternalTs=off  SampleTime=-1  IntegratorMethod=Forward Euler  FilterMethod=Forward Euler  ControllerParametersSource=internal  P=7  I=57.479  UseKiTs=off  D=10  N=100  UseFilter=on  TunerSelectOption=Transfer Function Based (PID Tuner App)  InitialConditionSource=internal  InitialConditionForIntegrator=0  InitialConditionForFilter=0  DifferentiatorICPrevScaledInput=0  ExternalReset=none  TrackingMode=off  Kt=1  LimitOutput=off  SatLimitsSource=internal  UpperSaturationLimit=inf  LowerSaturationLimit=-inf  LinearizeAsGain=on  AntiWindupMode=none  Kb=1  LimitIntegrator=off  UpperIntegratorSaturationLimit=inf  LowerIntegratorSaturationLimit=-inf  POutMin=[]  POutMax=[]  IOutMin=[]  IOutMax=[]  DOutMin=[]  DOutMax=[]  NOutMin=[]  NOutMax=[]  SumOutMin=[]  SumOutMax=[]  SaturationOutMin=[]  SaturationOutMax=[]  PParamMin=[]  PParamMax=[]  IParamMin=[]  IParamMax=[]  DParamMin=[]  DParamMax=[]  NParamMin=[]  NParamMax=[]  KbParamMin=[]  KbParamMax=[]  KtParamMin=[]  KtParamMax=[]  KbOutMin=[]  KbOutMax=[]  KtOutMin=[]  KtOutMax=[]  IntegratorOutMin=[]  IntegratorOutMax=[]  FilterOutMin=[]  FilterOutMax=[]  SumI1OutMin=[]  SumI1OutMax=[]  SumI2OutMin=[]  SumI2OutMax=[]  SumI3OutMin=[]  SumI3OutMax=[]  SumI4OutMin=[]  SumI4OutMax=[]  SumDOutMin=[]  SumDOutMax=[]  DifferentiatorOutMin=[]  DifferentiatorOutMax=[]  FilterDiffOutCoefMin=[]  FilterDiffOutCoefMax=[]  ReciprocalOutMin=[]  ReciprocalOutMax=[]  SumDenOutMin=[]  SumDenOutMax=[]  SumNumOutMin=[]  SumNumOutMax=[]  DivideOutMin=[]  DivideOutMax=[]  UdiffTsProdOutMin=[]  UdiffTsProdOutMax=[]  NTsProdOutMin=[]  NTsProdOutMax=[]  UintegralTsProdOutMin=[]  UintegralTsProdOutMax=[]  UngainTsProdOutMin=[]  UngainTsProdOutMax=[]  ClampingZeroOutDataTypeStr=Inherit: Inherit via back propagation  ClampingZeroOutMin=[]  ClampingZeroOutMax=[]  FilterDenConstantOutDataTypeStr=Inherit: Inherit via back propagation  FilterDenConstantOutMin=[]  FilterDenConstantOutMax=[]  PCopyOutDataTypeStr=Inherit: Inherit via back propagation  PCopyOutMin=[]  PCopyOutMax=[]  NCopyOutDataTypeStr=Inherit: Inherit via back propagation  NCopyOutMin=[]  NCopyOutMax=[]  IntegratorContinuousStateAttributes=''  IntegratorStateMustResolveToSignalObject=off  IntegratorRTWStateStorageClass=Auto  FilterContinuousStateAttributes=''  FilterStateMustResolveToSignalObject=off  FilterRTWStateStorageClass=Auto  ParallelPVariant=InternalParameters  IdealPVariant=Disabled  IVariant=Disabled  DVariant=InternalParameters  IntegratorVariant=Disabled  SatVariant=Disabled  AWVariant=Disabled  PCopyVariant=Disabled  TRVariant=Disabled  FdbkBlocksVariant=Forward  IdealPFdbkVariant=Disabled  SatFdbkVariant=Disabled  DerivativeFilterVariant=ContFilter  NVariant=InternalParameters  NCopyVariant=Disabled  FilterICVariant=InternalICsFilter  IntegratorICVariant=Disabled  ExternalResetVariant=Disabled  TRSumVariant=Passthrough  SumFdbkVariant=Disabled  SumVariant=Sum_PD  TsampFilterVariant=InternalTs  TsampNgainVariant=Passthrough  TsampIntegralVariant=Disabled_SignalSpec  ExternalSaturationOutDataTypeStr=Inherit: Same as second input
  Sum : Sum  Inputs=|+-
  delta_roll : Outport
  tag scope: phi_actual=global, phi_command=global
  wires:
  phi_command/1 -> Sum/1, [phi_command]
  Bus Selector/1 -> Sum/2, [phi_actual]  "<phi>"
  phi_actual/1 -> Bus Selector/1
  Sum/1 -> PID Controller1/1  "error"
  PID Controller1/1 -> delta_roll/1

== system untitled/Subsystem3/Subsystem5 ==
  note: X_theta_comm=X/theta * theta/theta_comm
      | X/ theta =-g/s^2
      | theta_comm=Kp(X_comm-X_actual)-Kd*X_dot
  x_command : Inport
  x_actual : Inport  Port=2
  Bus Selector : BusSelector  OutputSignals=X
  Derivative : Derivative
  Gain : Gain  Gain=0.15
  Gain1 : Gain  Gain=0.07
  Gain2 : Gain  Gain=-1
  Sum : Sum  Inputs=|+-
  Sum1 : Sum  Inputs=|+-
  theta_commanded : Outport
  tag scope: x_actual=global, x_command=global
  wires:
  x_command/1 -> Sum/1, [x_command]
  x_actual/1 -> Bus Selector/1
  Gain2/1 -> theta_commanded/1
  Bus Selector/1 -> Sum/2, Derivative/1, [x_actual]  "<X>"
  Gain/1 -> Sum1/2
  Sum/1 -> Gain1/1  "error"
  Derivative/1 -> Gain/1
  Sum1/1 -> Gain2/1
  Gain1/1 -> Sum1/1

== system untitled/Subsystem3/Subsystem6 ==
  y_command : Inport
  y_actual : Inport  Port=2
  Bus Selector : BusSelector  OutputSignals=Y
  Derivative : Derivative
  Gain : Gain  Gain=.13
  Gain1 : Gain  Gain=0.05
  Sum : Sum  Inputs=|+-
  Sum1 : Sum  Inputs=|+-
  phi_command : Outport
  tag scope: y_actual=global, y_command=global
  wires:
  y_actual/1 -> Bus Selector/1
  y_command/1 -> [y_command], Sum/1
  Gain1/1 -> Sum1/1
  Sum1/1 -> phi_command/1
  Derivative/1 -> Gain/1
  Sum/1 -> Gain1/1  "error"
  Gain/1 -> Sum1/2
  Bus Selector/1 -> [y_actual], Derivative/1, Sum/2  "<Y>"

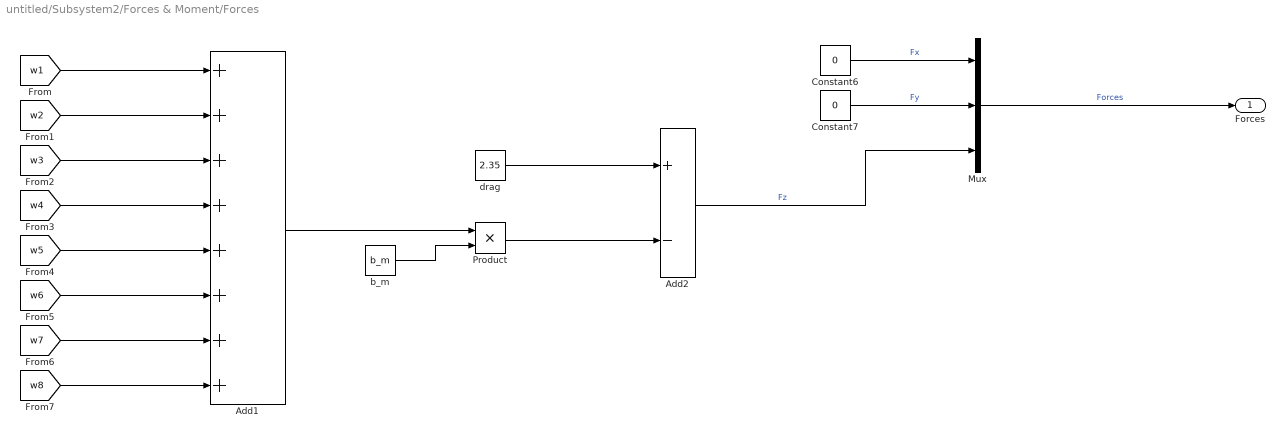
== system untitled/Subsystem2/Forces & Moment/Forces ==
  Add1 : Sum  Inputs=++++++++
  Add2 : Sum  Inputs=+-
  Constant6 : Constant  Value=0
  Constant7 : Constant  Value=0
  Mux : Mux  Inputs=3
  Product : Product
  b_m : Constant  Value=b_m
  drag : Constant  Value=2.35
  Forces : Outport
  wires:
  Constant6/1 -> Mux/1  "Fx"
  [w4] -> Add1/4
  b_m/1 -> Product/2
  Product/1 -> Add2/2
  [w8] -> Add1/8
  drag/1 -> Add2/1
  Add1/1 -> Product/1
  Constant7/1 -> Mux/2  "Fy"
  [w7] -> Add1/7
  [w2] -> Add1/2
  [w1] -> Add1/1
  [w6] -> Add1/6
  [w3] -> Add1/3
  [w5] -> Add1/5
  Add2/1 -> Mux/3  "Fz"
  Mux/1 -> Forces/1  "Forces"

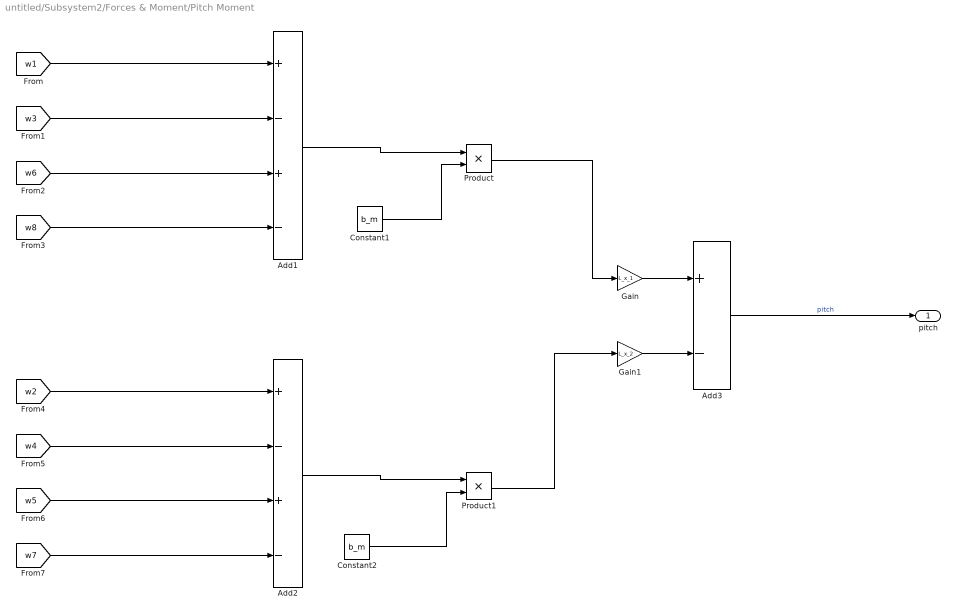
== system untitled/Subsystem2/Forces & Moment/Pitch Moment ==
  Add1 : Sum  Inputs=+-+-
  Add2 : Sum  Inputs=+-+-
  Add3 : Sum  Inputs=+-
  Constant1 : Constant  Value=b_m
  Constant2 : Constant  Value=b_m
  Gain : Gain  Gain=L_x_1
  Gain1 : Gain  Gain=L_x_2
  Product : Product
  Product1 : Product
  pitch : Outport
  wires:
  Add1/1 -> Product/1
  [w3] -> Add1/2
  Add3/1 -> pitch/1  "pitch"
  [w7] -> Add2/4
  [w5] -> Add2/3
  [w4] -> Add2/2
  Add2/1 -> Product1/1
  [w2] -> Add2/1
  [w1] -> Add1/1
  [w6] -> Add1/3
  [w8] -> Add1/4
  Product1/1 -> Gain1/1
  Product/1 -> Gain/1
  Constant1/1 -> Product/2
  Constant2/1 -> Product1/2
  Gain/1 -> Add3/1
  Gain1/1 -> Add3/2

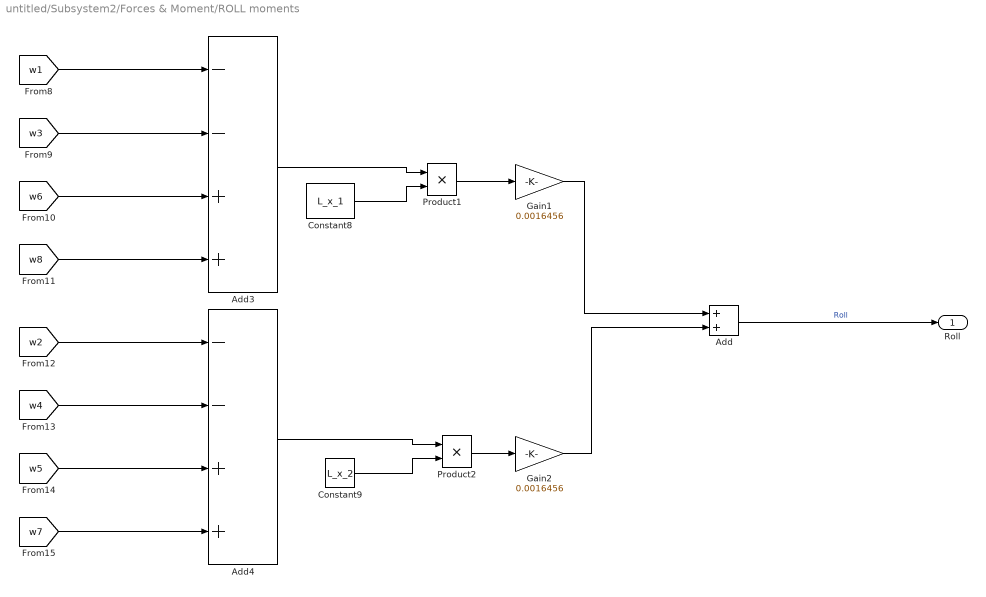
== system untitled/Subsystem2/Forces & Moment/ROLL moments ==
  Add : Sum
  Add3 : Sum  Inputs=--++
  Add4 : Sum  Inputs=--++
  Constant8 : Constant  Value=L_x_1
  Constant9 : Constant  Value=L_x_2
  Gain1 : Gain  Gain=0.0016456
  Gain2 : Gain  Gain=0.0016456
  Product1 : Product
  Product2 : Product
  Roll : Outport
  wires:
  [w5] -> Add4/3
  [w2] -> Add4/1
  [w7] -> Add4/4
  [w3] -> Add3/2
  Constant9/1 -> Product2/2
  [w1] -> Add3/1
  [w4] -> Add4/2
  [w8] -> Add3/4
  [w6] -> Add3/3
  Product1/1 -> Gain1/1
  Constant8/1 -> Product1/2
  Product2/1 -> Gain2/1
  Add/1 -> Roll/1  "Roll"
  Add3/1 -> Product1/1
  Add4/1 -> Product2/1
  Gain2/1 -> Add/2
  Gain1/1 -> Add/1

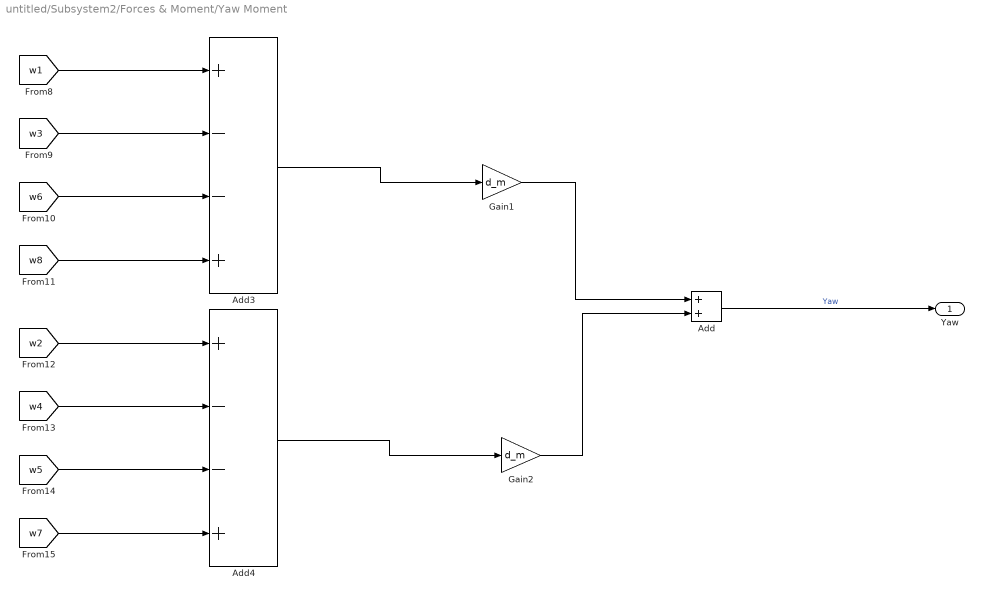
== system untitled/Subsystem2/Forces & Moment/Yaw Moment ==
  Add : Sum
  Add3 : Sum  Inputs=+--+
  Add4 : Sum  Inputs=+--+
  Gain1 : Gain  Gain=d_m
  Gain2 : Gain  Gain=d_m
  Yaw : Outport
  wires:
  Add/1 -> Yaw/1  "Yaw"
  Add4/1 -> Gain2/1
  Add3/1 -> Gain1/1
  [w6] -> Add3/3
  [w8] -> Add3/4
  [w4] -> Add4/2
  [w1] -> Add3/1
  [w3] -> Add3/2
  [w7] -> Add4/4
  [w2] -> Add4/1
  [w5] -> Add4/3
  Gain2/1 -> Add/2
  Gain1/1 -> Add/1

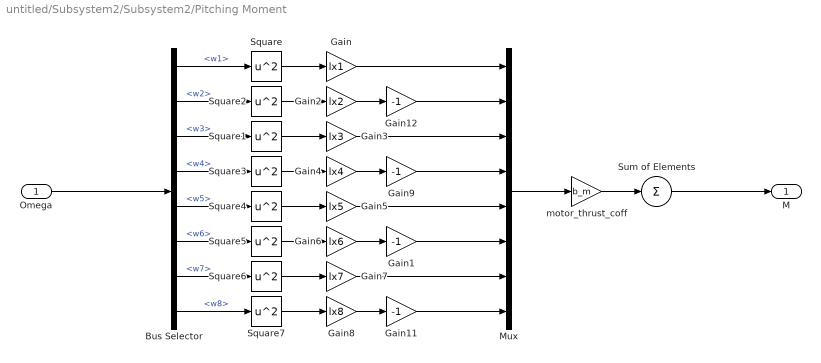
== system untitled/Subsystem2/Subsystem2/Pitching Moment ==
  Omega : Inport
  Bus Selector : BusSelector  OutputSignals=w1,w2,w3,w4,w5,w6,w7,w8
  Gain : Gain  Gain=lx1
  Gain{1,9,11..12} (4 alike) : Gain  Gain=-1
  Gain2 : Gain  Gain=lx2
  Gain3 : Gain  Gain=lx3
  Gain4 : Gain  Gain=lx4
  Gain5 : Gain  Gain=lx5
  Gain6 : Gain  Gain=lx6
  Gain7 : Gain  Gain=lx7
  Gain8 : Gain  Gain=lx8
  Mux : Mux  Inputs=8
  Square{,1..7} (8 alike) : Math  Operator=square
  Sum of Elements : Sum  Inputs=+
  motor_thrust_coff : Gain  Gain=b_m
  M : Outport
  wires:
  motor_thrust_coff/1 -> Sum of Elements/1
  Square4/1 -> Gain5/1
  Gain3/1 -> Mux/3
  Bus Selector/2 -> Square2/1  "<w2>"
  Bus Selector/6 -> Square5/1  "<w6>"
  Bus Selector/8 -> Square7/1  "<w8>"
  Gain6/1 -> Gain1/1
  Gain/1 -> Mux/1
  Gain11/1 -> Mux/8
  Gain4/1 -> Gain9/1
  Gain2/1 -> Gain12/1
  Bus Selector/1 -> Square/1  "<w1>"
  Bus Selector/5 -> Square4/1  "<w5>"
  Square5/1 -> Gain6/1
  Square7/1 -> Gain8/1
  Gain7/1 -> Mux/7
  Square/1 -> Gain/1
  Bus Selector/4 -> Square3/1  "<w4>"
  Gain8/1 -> Gain11/1
  Bus Selector/7 -> Square6/1  "<w7>"
  Gain5/1 -> Mux/5
  Bus Selector/3 -> Square1/1  "<w3>"
  Mux/1 -> motor_thrust_coff/1
  Square6/1 -> Gain7/1
  Sum of Elements/1 -> M/1
  Square3/1 -> Gain4/1
  Square2/1 -> Gain2/1
  Gain9/1 -> Mux/4
  Square1/1 -> Gain3/1
  Omega/1 -> Bus Selector/1
  Gain12/1 -> Mux/2
  Gain1/1 -> Mux/6

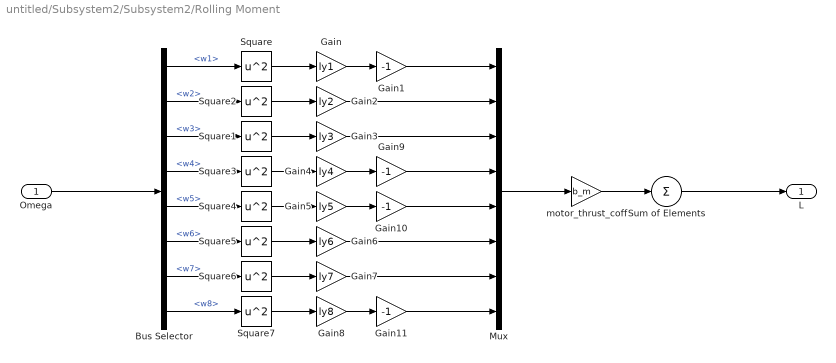
== system untitled/Subsystem2/Subsystem2/Rolling Moment ==
  Omega : Inport
  Bus Selector : BusSelector  OutputSignals=w1,w2,w3,w4,w5,w6,w7,w8
  Gain : Gain  Gain=ly1
  Gain{1,9..11} (4 alike) : Gain  Gain=-1
  Gain2 : Gain  Gain=ly2
  Gain3 : Gain  Gain=ly3
  Gain4 : Gain  Gain=ly4
  Gain5 : Gain  Gain=ly5
  Gain6 : Gain  Gain=ly6
  Gain7 : Gain  Gain=ly7
  Gain8 : Gain  Gain=ly8
  Mux : Mux  Inputs=8
  Square{,1..7} (8 alike) : Math  Operator=square
  Sum of Elements : Sum  Inputs=+
  motor_thrust_coff : Gain  Gain=b_m
  L : Outport
  wires:
  Omega/1 -> Bus Selector/1
  Bus Selector/1 -> Square/1  "<w1>"
  Square/1 -> Gain/1
  Gain/1 -> Gain1/1
  Bus Selector/3 -> Square1/1  "<w3>"
  Bus Selector/2 -> Square2/1  "<w2>"
  Bus Selector/4 -> Square3/1  "<w4>"
  Bus Selector/5 -> Square4/1  "<w5>"
  Bus Selector/6 -> Square5/1  "<w6>"
  Bus Selector/7 -> Square6/1  "<w7>"
  Bus Selector/8 -> Square7/1  "<w8>"
  Square2/1 -> Gain2/1
  Square1/1 -> Gain3/1
  Square3/1 -> Gain4/1
  Square4/1 -> Gain5/1
  Square5/1 -> Gain6/1
  Square6/1 -> Gain7/1
  Square7/1 -> Gain8/1
  Gain4/1 -> Gain9/1
  Gain5/1 -> Gain10/1
  Gain8/1 -> Gain11/1
  Gain1/1 -> Mux/1
  Gain2/1 -> Mux/2
  Gain3/1 -> Mux/3
  Gain9/1 -> Mux/4
  Gain10/1 -> Mux/5
  Gain6/1 -> Mux/6
  Gain7/1 -> Mux/7
  Gain11/1 -> Mux/8
  Mux/1 -> motor_thrust_coff/1
  Sum of Elements/1 -> L/1
  motor_thrust_coff/1 -> Sum of Elements/1

== system untitled/Subsystem2/Subsystem2/Subsystem ==
  omegas : Inport
  Add : Sum  Inputs=++++++++
  Bus Selector : BusSelector  OutputSignals=w1,w2,w3,w4,w5,w6,w7,w8
  Square{,1..7} (8 alike) : Math  Operator=square
  motor_thrust_coff : Gain  Gain=b_m
  Fz : Outport
  wires:
  omegas/1 -> Bus Selector/1
  Bus Selector/1 -> Square/1  "<w1>"
  Bus Selector/6 -> Square5/1  "<w6>"
  Bus Selector/2 -> Square1/1  "<w2>"
  Bus Selector/3 -> Square2/1  "<w3>"
  Bus Selector/4 -> Square3/1  "<w4>"
  Bus Selector/5 -> Square4/1  "<w5>"
  Bus Selector/7 -> Square6/1  "<w7>"
  Bus Selector/8 -> Square7/1  "<w8>"
  Add/1 -> motor_thrust_coff/1
  motor_thrust_coff/1 -> Fz/1
  Square/1 -> Add/1
  Square1/1 -> Add/2
  Square2/1 -> Add/3
  Square3/1 -> Add/4
  Square4/1 -> Add/5
  Square5/1 -> Add/6
  Square6/1 -> Add/7
  Square7/1 -> Add/8

== system untitled/Subsystem2/Subsystem2/Subsystem1 ==
  Omegas : Inport
  Bus Creator1 : BusCreator  Inputs=8
  Demux : Demux  Outputs=8
  Omega : Outport
  wires:
  Demux/7 -> Bus Creator1/7  "w7"
  Demux/3 -> Bus Creator1/3  "w3"
  Demux/2 -> Bus Creator1/2  "w2"
  Demux/4 -> Bus Creator1/4  "w4"
  Demux/5 -> Bus Creator1/5  "w5"
  Demux/6 -> Bus Creator1/6  "w6"
  Demux/1 -> Bus Creator1/1  "w1"
  Demux/8 -> Bus Creator1/8  "w8"
  Bus Creator1/1 -> Omega/1
  Omegas/1 -> Demux/1

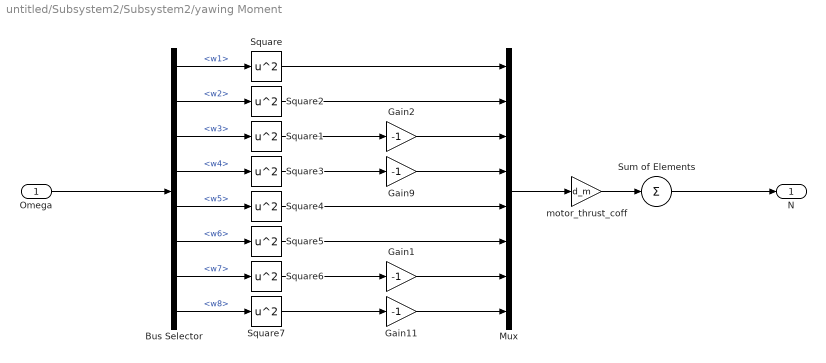
== system untitled/Subsystem2/Subsystem2/yawing Moment ==
  Omega : Inport
  Bus Selector : BusSelector  OutputSignals=w1,w2,w3,w4,w5,w6,w7,w8
  Gain{1..2,9,11} (4 alike) : Gain  Gain=-1
  Mux : Mux  Inputs=8
  Square{,1..7} (8 alike) : Math  Operator=square
  Sum of Elements : Sum  Inputs=+
  motor_thrust_coff : Gain  Gain=d_m
  N : Outport
  wires:
  Square2/1 -> Mux/2
  Gain9/1 -> Mux/4
  Bus Selector/3 -> Square1/1  "<w3>"
  Mux/1 -> motor_thrust_coff/1
  Bus Selector/5 -> Square4/1  "<w5>"
  Bus Selector/1 -> Square/1  "<w1>"
  Square6/1 -> Gain1/1
  Square7/1 -> Gain11/1
  Square5/1 -> Mux/6
  Bus Selector/7 -> Square6/1  "<w7>"
  Bus Selector/4 -> Square3/1  "<w4>"
  Square3/1 -> Gain9/1
  Square1/1 -> Gain2/1
  Bus Selector/8 -> Square7/1  "<w8>"
  motor_thrust_coff/1 -> Sum of Elements/1
  Gain11/1 -> Mux/8
  Bus Selector/6 -> Square5/1  "<w6>"
  Bus Selector/2 -> Square2/1  "<w2>"
  Square/1 -> Mux/1
  Square4/1 -> Mux/5
  Omega/1 -> Bus Selector/1
  Sum of Elements/1 -> N/1
  Gain2/1 -> Mux/3
  Gain1/1 -> Mux/7

== matlab function untitled/Subsystem2/Forces & Moment/MATLAB Function ==
  data: omegas input size=[8,1]; D input; L input; ceta input; F output size=[1,3]; b_m input; d_m input; lx1 input; lx2 input; lx3 input; M output; lx4 input; lx5 input; lx6 input; lx7 input; lx8 input; ly1 input; ly2 input; ly3 input; ly4 input; ly5 input; ly6 input; ly7 input; ly8 input
function [F,M] = fcn(omegas,D,L,ceta, b_m,d_m,lx1,lx2, lx3, lx4, lx5, lx6, lx7, lx8, ly1, ly2, ly3, ly4, ly5, ly6, ly7, ly8)
w1=omegas(1);
w2=omegas(2);
w3=omegas(3);
w4=omegas(4);
w5=omegas(5);
w6=omegas(6);
w7=omegas(7);
w8=omegas(8);

Fx=0;
Fy=0;                            % Aerodynamic force needed 
Fz=-b_m*(w1^2+w2^2+w3^2+w4^2+w5^2+w6^2+w7^2+w8^2);                        % Aerodynamic force needed 
L_roll=(b_m*(-ly1*w1^2-ly4*w4^2-ly5*w5^2-ly8*w8^2))+(b_m)*(ly3*w3^2+ly2*w2^2+ly7*w7^2+ly6*w6^2);
M_Pitch=(b_m*(lx1*w1^2+lx3*w3^2+lx5*w5^2+lx7*w7^2))+(b_m*(-lx2*w2^2-lx4*w4^2-lx6*w6^2-lx8*w8^2));
N_yaw=d_m*((w1^2+w2^2+w5^2+w6^2)-(w3^2+w4^2+w7^2+w8^2));

F=[Fx Fy Fz];
M=[L_roll  M_Pitch N_yaw];

== matlab function untitled/Subsystem2/Forces & Moment/MATLAB Function1 ==
  data: omegas input size=[8,1]; D input; L input; ceta input; F output size=[1,3]; b_m input; d_m input; l_1 input; l_2 input; M output
function [F,M] = fcn(omegas,D,L,ceta, b_m,d_m,l_1,l_2)
w1=omegas(1);
w2=omegas(2);
w3=omegas(3);
w4=omegas(4);
w5=omegas(5);
w6=omegas(6);
w7=omegas(7);
w8=omegas(8);
F_F_z=b_m*(w1^2+w2^2+w6^2+w5^2)+b_m*(w8^2+w7^2+w4^2+w3^2);

Fx=0;
Fy=0;                            % Aerodynamic force needed 
Fz=D-F_F_z;                        % Aerodynamic force needed 
L_roll=(b_m*l_1*(-w1^2-w3^2+w6^2+w8^2))+(b_m*l_2)*(-w2^2-w4^2+w7^2+w5^2);
M_Pitch=(b_m*l_1*(w1^2-w3^2+w6^2-w8^2))+(b_m*l_2*(w2^2-w4^2+w5^2-w7^2));
 N_yaw=(d_m*l_1*(w1^2-w3^2+w8^2-w6^2))+(d_m*l_2*(w2^2-w4^2+w7^2-w5^2));

F=[Fx Fy Fz];
M=[L_roll  M_Pitch N_yaw];
